simulink model "edo"  (R2023a)
settings: Solver=FixedStepAuto  StartTime=0.0  StopTime=10  FixedStep=0.01  RelTol=1e-3
undefined symbols (not defined in the file): g, K, l
settings Model: PacingRate=0.100000  Creator=ave9761  LastModifiedBy=ave9761

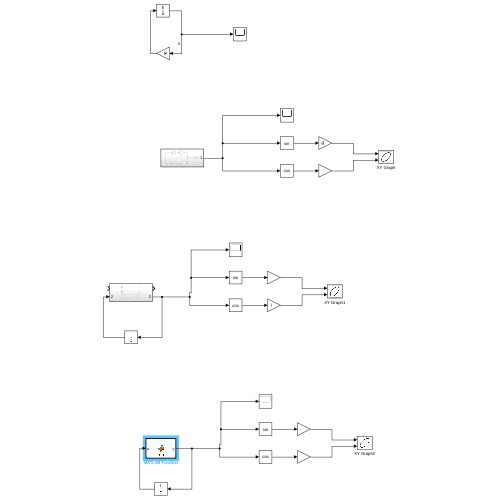
[thumbnail: Simulink's stored preview of the top-level diagram]
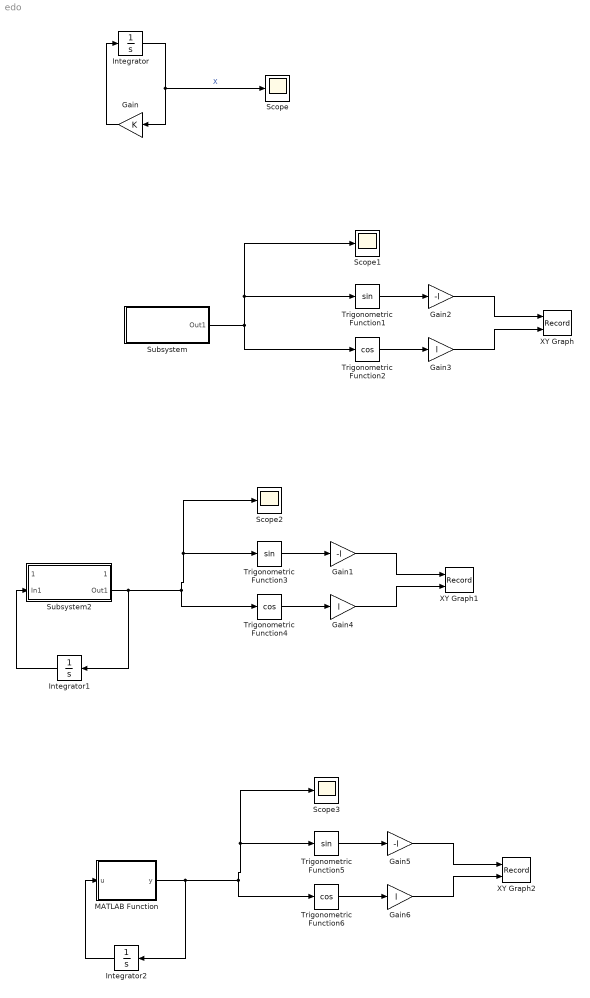
== system edo ==
  Gain : Gain  Gain=K
  Gain1 : Gain  Gain=-l
  Gain2 : Gain  Gain=-l
  Gain3 : Gain  Gain=l
  Gain4 : Gain  Gain=l
  Gain5 : Gain  Gain=-l
  Gain6 : Gain  Gain=l
  Integrator : Integrator  InitialCondition=1
  Integrator1 : Integrator
  Integrator2 : Integrator
  MATLAB Function : MATLAB Function  TreatAsAtomicUnit=on
  Scope{,1..3} (4 alike) : Scope
  Subsystem : Subsystem
  Subsystem2 : Subsystem
  Trigonometric Function1 : Trigonometry
  Trigonometric Function2 : Trigonometry  Operator=cos
  Trigonometric Function3 : Trigonometry
  Trigonometric Function4 : Trigonometry  Operator=cos
  Trigonometric Function5 : Trigonometry
  Trigonometric Function6 : Trigonometry  Operator=cos
  XY Graph : Record  FileSettingsInternal="{\"entries\":[{\"content\":{\"excelSettings\":{\"content\":{},\"type\":\"Streamout.ExcelSettings\"}},\"type\":\"Streamout.FileSettingStorage\",\"uuid\":\"e74e9f9a-8702-4627-b676-2e0f7d5adedc\"}],\"packageUris\":[\"http://schema.mathworks.com/mf0/streamout_blocks/R2020a\"],\"version\":\"1.0\"}"  Layout=[1 1]  SignalsInternal="{\"entries\":[{\"content\":{\"signals\":[{\"content\":{\"blockPath\":[\"edo/XY Graph\"],\"dimensions\":[1],\"domain\":\"edo/XY Graph\",\"lineColor\":\"#a2142f\",\"plots\":[1],\"port\":1,\"sid\":[\"\"],\"signalID\":281,\"signalName\":\"Gain2\"},\"type\":\"RecordBlkView.Signal\",\"uuid\":\"3cea4adf-1f31-4f43-bdb6-e9d4b6e186fb\"},{\"content\":{\"blockPath\":[\"edo/XY Graph\"],\"dimensions\":[1],\"domain\":\"edo/XY Graph\",\"lineColor\":\"#139fff\",\"plots\":[1],\"port\":2,\"sid\":[\"\"],\"signalID\":285,\"signalName\":\"Gain3\"},\"type\":\"RecordBlkView.Signal\",\"uuid\":\"f7f7d996-de59-4f4a-b1e4-f1c5e84fa885\"}]},\"type\":\"RecordBlkView.InputSignals\",\"uuid\":\"6e4b4115-ae48-42d5-a589-05dcef9a5491\"}],\"packageUris\":[\"http://schema.mathworks.com/mf0/streamout_blocks/R2020a\"],\"version\":\"1.0\"}"  VisualizationBindings="{\"xyplotplugin\":{\"info\":[{\"series\":[{\"bindingParametersList\":[{\"parameter\":\"X-Axis\",\"signalID\":281,\"signalName\":\"Gain2\"},{\"parameter\":\"Y-Axis\",\"signalID\":285,\"signalName\":\"Gain3\"}],\"seriesID\":11878}],\"subplotID\":1}]}}"  CompatibilityTag=XY
  XY Graph1 : Record  FileSettingsInternal="{\"entries\":[{\"content\":{\"excelSettings\":{\"content\":{},\"type\":\"Streamout.ExcelSettings\"}},\"type\":\"Streamout.FileSettingStorage\",\"uuid\":\"dcb174fb-1fb4-4ae2-8074-f93479a1f593\"}],\"packageUris\":[\"http://schema.mathworks.com/mf0/streamout_blocks/R2020a\"],\"version\":\"1.0\"}"  Layout=[1 1]  SignalsInternal="{\"entries\":[{\"content\":{\"signals\":[{\"content\":{\"blockPath\":[\"edo/XY Graph1\"],\"dimensions\":[1],\"domain\":\"edo/XY Graph1\",\"lineColor\":\"#a2142f\",\"plots\":[1],\"port\":1,\"signalID\":300,\"signalName\":\"XY Graph:1\"},\"type\":\"RecordBlkView.Signal\",\"uuid\":\"02e61dfe-b87e-4a1b-a190-ccbc527817cb\"},{\"content\":{\"blockPath\":[\"edo/XY Graph1\"],\"dimensions\":[1],\"domain\":\"edo/XY Graph1\",\"lineColor\":\"#139fff\",\"plots\":[1],\"port\":2,\"signalID\":303,\"signalName\":\"XY Graph:2\"},\"type\":\"RecordBlkView.Signal\",\"uuid\":\"886dcf3d-3f84-406b-b53a-6a46e03f8e5c\"}]},\"type\":\"RecordBlkView.InputSignals\",\"uuid\":\"1785c29c-fa33-4f63-87cf-8ab461bf8a29\"}],\"packageUris\":[\"http://schema.mathworks.com/mf0/streamout_blocks/R2020a\"],\"version\":\"1.0\"}"  VisualizationBindings="{\"xyplotplugin\":{\"info\":[{\"series\":[{\"bindingParametersList\":[{\"parameter\":\"X-Axis\",\"signalID\":300,\"signalName\":\"XY Graph:1\"},{\"parameter\":\"Y-Axis\",\"signalID\":303,\"signalName\":\"XY Graph:2\"}],\"seriesID\":58980}],\"subplotID\":1}]}}"  CompatibilityTag=XY
  XY Graph2 : Record  FileSettingsInternal="{\"entries\":[{\"content\":{\"excelSettings\":{\"content\":{},\"type\":\"Streamout.ExcelSettings\"}},\"type\":\"Streamout.FileSettingStorage\",\"uuid\":\"5a1ad372-d3c1-4ca5-8f0e-201427a122a8\"}],\"packageUris\":[\"http://schema.mathworks.com/mf0/streamout_blocks/R2020a\"],\"version\":\"1.0\"}"  Layout=[1 1]  SignalsInternal="{\"entries\":[{\"content\":{\"signals\":[{\"content\":{\"blockPath\":[\"edo/XY Graph2\"],\"dimensions\":[1],\"domain\":\"edo/XY Graph2\",\"lineColor\":\"#a2142f\",\"plots\":[1],\"port\":1,\"signalID\":308,\"signalName\":\"XY Graph:1\"},\"type\":\"RecordBlkView.Signal\",\"uuid\":\"d64bf269-6a66-4b2b-b840-6cc7df120b46\"},{\"content\":{\"blockPath\":[\"edo/XY Graph2\"],\"dimensions\":[1],\"domain\":\"edo/XY Graph2\",\"lineColor\":\"#139fff\",\"plots\":[1],\"port\":2,\"signalID\":311,\"signalName\":\"XY Graph:2\"},\"type\":\"RecordBlkView.Signal\",\"uuid\":\"c552787e-0b86-456e-a6d6-118ded65fa8b\"}]},\"type\":\"RecordBlkView.InputSignals\",\"uuid\":\"bde78419-3fb4-4d33-8e04-cbe7c8ff28f8\"}],\"packageUris\":[\"http://schema.mathworks.com/mf0/streamout_blocks/R2020a\"],\"version\":\"1.0\"}"  VisualizationBindings="{\"xyplotplugin\":{\"info\":[{\"series\":[{\"bindingParametersList\":[{\"parameter\":\"X-Axis\",\"signalID\":308,\"signalName\":\"XY Graph:1\"},{\"parameter\":\"Y-Axis\",\"signalID\":311,\"signalName\":\"XY Graph:2\"}],\"seriesID\":52508}],\"subplotID\":1}]}}"  CompatibilityTag=XY
  wires:
  Gain/1 -> Integrator/1
  Integrator/1 -> Scope/1, Gain/1  "X"
  Trigonometric Function1/1 -> Gain2/1
  Trigonometric Function2/1 -> Gain3/1
  Gain2/1 -> XY Graph/1
  Gain3/1 -> XY Graph/2
  Subsystem/1(Out1) -> Trigonometric Function1/1, Scope1/1, Trigonometric Function2/1
  Trigonometric Function4/1 -> Gain4/1
  Trigonometric Function3/1 -> Gain1/1
  Gain1/1 -> XY Graph1/1
  Subsystem2/2(Out1) -> Integrator1/1, Trigonometric Function3/1, Scope2/1, Trigonometric Function4/1
  Gain4/1 -> XY Graph1/2
  Integrator1/1 -> Subsystem2/2(In1)
  Trigonometric Function5/1 -> Gain5/1
  Gain5/1 -> XY Graph2/1
  Integrator2/1 -> MATLAB Function/1(u)
  Gain6/1 -> XY Graph2/2
  Trigonometric Function6/1 -> Gain6/1
  MATLAB Function/1(y) -> Integrator2/1, Trigonometric Function5/1, Scope3/1, Trigonometric Function6/1

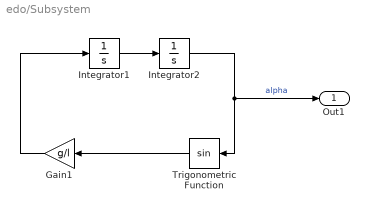
== system edo/Subsystem ==
  Gain1 : Gain  Gain=g/l
  Integrator1 : Integrator
  Integrator2 : Integrator  InitialCondition=1
  Trigonometric Function : Trigonometry
  Out1 : Outport
  wires:
  Integrator1/1 -> Integrator2/1
  Trigonometric Function/1 -> Gain1/1
  Gain1/1 -> Integrator1/1
  Integrator2/1 -> Out1/1, Trigonometric Function/1  "alpha"

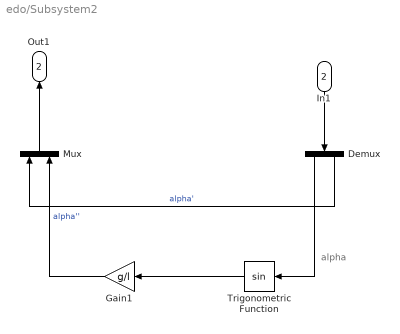
== system edo/Subsystem2 ==
  note: alpha
  In1 : Inport  Port=2
  Demux : Demux  Outputs=2
  Gain1 : Gain  Gain=g/l
  Mux : Mux  Inputs=2
  Trigonometric Function : Trigonometry
  Out1 : Outport  Port=2
  wires:
  Trigonometric Function/1 -> Gain1/1
  Gain1/1 -> Mux/2  "alpha''"
  Demux/2 -> Mux/1  "alpha'"
  Demux/1 -> Trigonometric Function/1
  Mux/1 -> Out1/1
  In1/1 -> Demux/1

== matlab function edo/MATLAB Function ==
  data: u input; y output
function y = fcn(u)

y = [  ];
